simulink model "reaction_wheels_design_v03"  (R2015b)
settings: Solver=VariableStepAuto  StartTime=0.0  StopTime=stop_time  RelTol=1e-6
values from neighbouring files (symbols this model uses):
  I_x = 1    [main_linear_spacecraft_euler.m]    (also in main_reaction_nonlinear_v02.m; main_reaction_wheels_detumbling.m; main_reaction_wheels_nonlinear_v01.m; main_reaction_wheels_nonlinear_v03.m)
  I_y = 0.5    [main_linear_spacecraft_euler.m]    (also in main_reaction_nonlinear_v02.m; main_reaction_wheels_detumbling.m; main_reaction_wheels_nonlinear_v01.m; main_reaction_wheels_nonlinear_v03.m)
  I_z = 0.7    [main_linear_spacecraft_euler.m]    (also in main_reaction_nonlinear_v02.m; main_reaction_wheels_detumbling.m; main_reaction_wheels_nonlinear_v01.m; main_reaction_wheels_nonlinear_v03.m)
  omega_x_0 = 0    [main_linear_spacecraft_euler.m]    (also in main_reaction_wheels_detumbling.m = 0.02; main_reaction_wheels_nonlinear_v03.m)
  omega_y_0 = 0    [main_linear_spacecraft_euler.m]    (also in main_reaction_wheels_detumbling.m = 0.02; main_reaction_wheels_nonlinear_v03.m)
  omega_z_0 = 0    [main_linear_spacecraft_euler.m]    (also in main_reaction_wheels_detumbling.m = -0.03; main_reaction_wheels_nonlinear_v03.m)
  phi_0 = 0    [main_linear_spacecraft_euler.m]    (also in main_reaction_wheels_nonlinear_v03.m = 0.698131700798)
  psi_0 = 0    [main_linear_spacecraft_euler.m]    (also in main_reaction_wheels_nonlinear_v03.m = -1.0471975512)
  theta_0 = 0    [main_linear_spacecraft_euler.m]    (also in main_pd_control.m = 2; main_reaction_wheels_nonlinear_v03.m = -0.698131700798)
undefined symbols (not defined in the file or in its folder): k_d_x, k_d_y, k_d_z, k_p_x, k_p_y, k_p_z
settings Model: Creator=Krunal's PC  LastModifiedBy=Krunal's PC

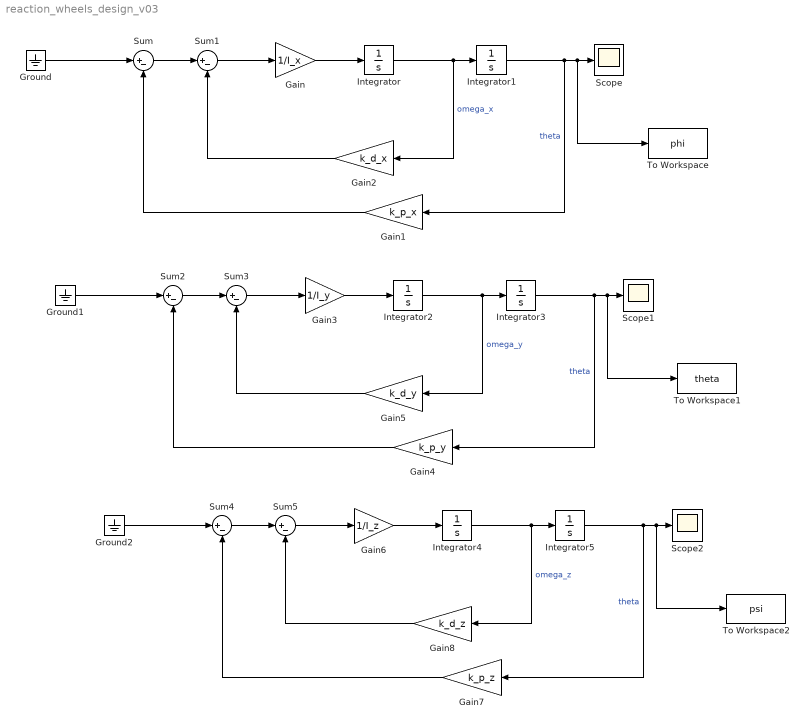
== system reaction_wheels_design_v03 ==
  Gain : Gain  Gain=1/I_x
  Gain1 : Gain  Gain=k_p_x
  Gain2 : Gain  Gain=k_d_x
  Gain3 : Gain  Gain=1/I_y
  Gain4 : Gain  Gain=k_p_y
  Gain5 : Gain  Gain=k_d_y
  Gain6 : Gain  Gain=1/I_z
  Gain7 : Gain  Gain=k_p_z
  Gain8 : Gain  Gain=k_d_z
  Ground : Ground
  Ground1 : Ground
  Ground2 : Ground
  Integrator : Integrator  InitialCondition=omega_x_0
  Integrator1 : Integrator  InitialCondition=phi_0
  Integrator2 : Integrator  InitialCondition=omega_y_0
  Integrator3 : Integrator  InitialCondition=theta_0
  Integrator4 : Integrator  InitialCondition=omega_z_0
  Integrator5 : Integrator  InitialCondition=psi_0
  Scope : Scope
  Scope1 : Scope
  Scope2 : Scope
  Sum{,1..5} (6 alike) : Sum  Inputs=|+-
  To Workspace : ToWorkspace  VariableName=phi  SampleTime=-1
  To Workspace1 : ToWorkspace  VariableName=theta  SampleTime=-1
  To Workspace2 : ToWorkspace  VariableName=psi  SampleTime=-1
  wires:
  Sum/1 -> Sum1/1
  Sum1/1 -> Gain/1
  Gain/1 -> Integrator/1
  Integrator/1 -> Gain2/1, Integrator1/1  "omega_x"
  Integrator1/1 -> Gain1/1, To Workspace/1, Scope/1  "theta"
  Gain1/1 -> Sum/2
  Gain2/1 -> Sum1/2
  Ground/1 -> Sum/1
  Sum2/1 -> Sum3/1
  Sum3/1 -> Gain3/1
  Gain3/1 -> Integrator2/1
  Integrator2/1 -> Integrator3/1, Gain5/1  "omega_y"
  Integrator3/1 -> Scope1/1, To Workspace1/1, Gain4/1  "theta"
  Gain4/1 -> Sum2/2
  Gain5/1 -> Sum3/2
  Ground1/1 -> Sum2/1
  Sum4/1 -> Sum5/1
  Sum5/1 -> Gain6/1
  Gain6/1 -> Integrator4/1
  Integrator4/1 -> Gain8/1, Integrator5/1  "omega_z"
  Integrator5/1 -> Gain7/1, To Workspace2/1, Scope2/1  "theta"
  Gain7/1 -> Sum4/2
  Gain8/1 -> Sum5/2
  Ground2/1 -> Sum4/1
